simulink model "main_controller_sim"  (R2015a)
settings: Solver=ode45  StartTime=0.0  StopTime=10  FixedStep=1e-4  MaxStep=1e-3  RelTol=1e-3
values from neighbouring files (symbols this model uses):
  A = [-1.27797343778 0.333872204357 1.75620734089 -1.56224484389 -1.03731554325 1.61047691587 -0.301778945187 -0.746429865998 -1.0138823557 1.30543582149 -0.0889326780489 0.0332636291631 ... (36 elements, 6x6)]    [A.mat]    (also in main_Observer.m = sys_rand.A)
  B = [-0.333073072673  -0.110223384653; -0.886176721199  0.948351131026; -0.150737126395  1.10111498524; 0  0.325274480302; 1.26534516191  1.00523432387; 0  0]    [B.mat]    (also in main_Observer.m = B(:,1:end-1))
  C = [0.8954663563 -0.344571536199 -1.3867839766 0 0 -1.25274492024 0.0740580691775 -0.828704014931 -0.552438671582 0 -0.23750602142 -0.378709097599 ... (18 elements, 3x6)]    [C.mat]    (also in main_Observer.m = sys_rand.C)
  Delta = (eye(n,n)+(-H*CHp+Y*(eye(p,p)-(C*H)*CHp))*C)*B    [main_Observer.m]    (also in observer.mat = [1.06190567075  -3.812249351; 850.258941028  448.332221539; )
  Gama = eta*A-X*C    [main_Observer.m]    (also in observer.mat = [22.8246151403 -1331.98593789 -219.710031357 145.030296815 2)
  H = [0.574066719729 0.519875550069 -0.636819062075 -0.770886938571 0.309777205751 -0.804844094201]    [H.mat]    (also in main_Observer.m = B(:,end))
  Phi = inv(delta1)*Phi_hat    [main_Observer.m]    (also in observer.mat = [35.9769844985 416.30041215 22.0641801854 39.341911218 -79.7)
  theta = theta1+Y*theta2    [main_Observer.m]    (also in observer.mat = [0.23961688316 -297.740368665 3.95476908974 -0.24732331029 -)
undefined symbols (not defined in the file or in its folder): beta, Tw, Tx
settings Model: Creator=p4wp4w  LastModifiedBy=p4wp4w

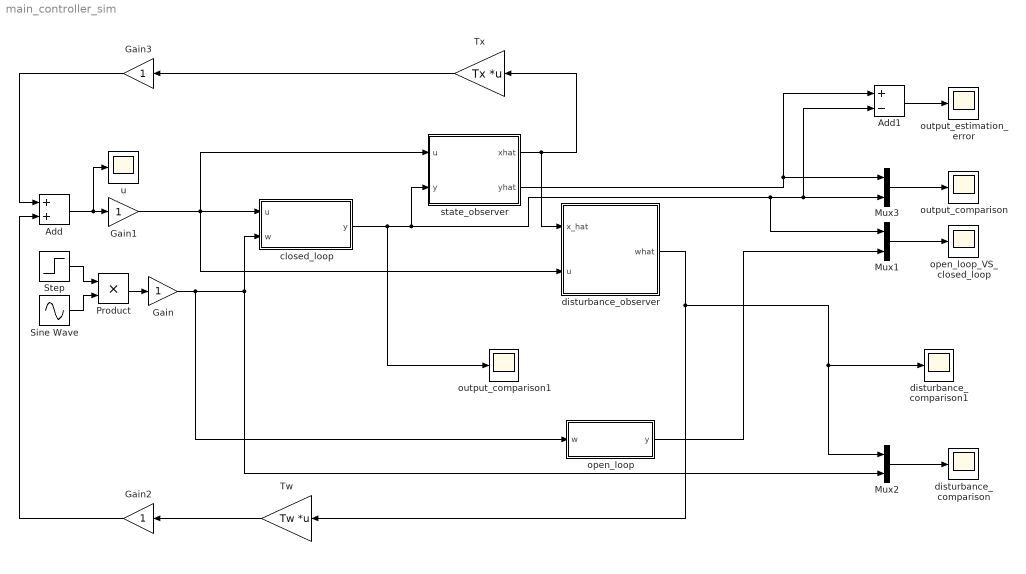
== system main_controller_sim ==
  Add : Sum
  Add1 : Sum  Inputs=+-
  Gain{,1..3} (4 alike) : Gain
  Mux1 : Mux  Inputs=2
  Mux2 : Mux  Inputs=2
  Mux3 : Mux  Inputs=2
  Product : Product
  Sine Wave : Sin  Frequency=10  SampleTime=0
  Step : Step  Before=8  After=0  SampleTime=0
  Tw : Gain  Gain=Tw  Multiplication=Matrix(K*u)
  Tx : Gain  Gain=Tx  Multiplication=Matrix(K*u)
  closed_loop : Subsystem
  disturbance_comparison : Scope
      settings: YMin=-15  YMax=15
  disturbance_comparison1 : Scope
      settings: YMin=-15  YMax=15  SaveName=ScopeData6
  disturbance_observer : Subsystem
  open_loop : Subsystem
  open_loop_VS_closed_loop : Scope
      settings: ShowLegends=on  YMin=-5e+22  YMax=3.5e+23  SaveName=ScopeData4
  output_comparison : Scope
      settings: YMin=-0.0024  YMax=-2.1684e-19
  output_comparison1 : Scope
      settings: YMin=-0.0024  YMax=-2.1684e-19  SaveName=ScopeData5
  output_estimation_error : Scope
      settings: YMin=-0.0024  YMax=-2.1684e-19  SaveName=ScopeData3
  state_observer : Subsystem
  u : Scope
      settings: SaveName=ScopeData2
  wires:
  Gain1/1 -> disturbance_observer/2(u), state_observer/1(u), closed_loop/1(u)
  closed_loop/1(y) -> output_comparison1/1, Mux1/1, Add1/2, Mux3/2, state_observer/2(y)
  Mux2/1 -> disturbance_comparison/1
  Mux3/1 -> output_comparison/1
  state_observer/2(yhat) -> Add1/1, Mux3/1
  disturbance_observer/1(what) -> Tw/1, disturbance_comparison1/1, Mux2/1
  Gain/1 -> open_loop/1(w), Mux2/2, closed_loop/2(w)
  state_observer/1(xhat) -> disturbance_observer/1(x_hat), Tx/1
  Add/1 -> u/1, Gain1/1
  Tx/1 -> Gain3/1
  Tw/1 -> Gain2/1
  Gain2/1 -> Add/2
  Gain3/1 -> Add/1
  Add1/1 -> output_estimation_error/1
  open_loop/1(y) -> Mux1/2
  Mux1/1 -> open_loop_VS_closed_loop/1
  Product/1 -> Gain/1
  Step/1 -> Product/1
  Sine Wave/1 -> Product/2

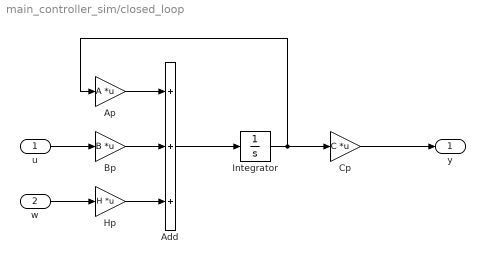
== system main_controller_sim/closed_loop ==
  u : Inport
  w : Inport  Port=2
  Add : Sum  Inputs=+++
  Ap : Gain  Gain=A  Multiplication=Matrix(K*u)
  Bp : Gain  Gain=B  Multiplication=Matrix(K*u)
  Cp : Gain  Gain=C  Multiplication=Matrix(K*u)
  Hp : Gain  Gain=H  Multiplication=Matrix(K*u)
  Integrator : Integrator
  y : Outport
  wires:
  w/1 -> Hp/1
  u/1 -> Bp/1
  Add/1 -> Integrator/1
  Bp/1 -> Add/2
  Integrator/1 -> Cp/1, Ap/1
  Ap/1 -> Add/1
  Hp/1 -> Add/3
  Cp/1 -> y/1

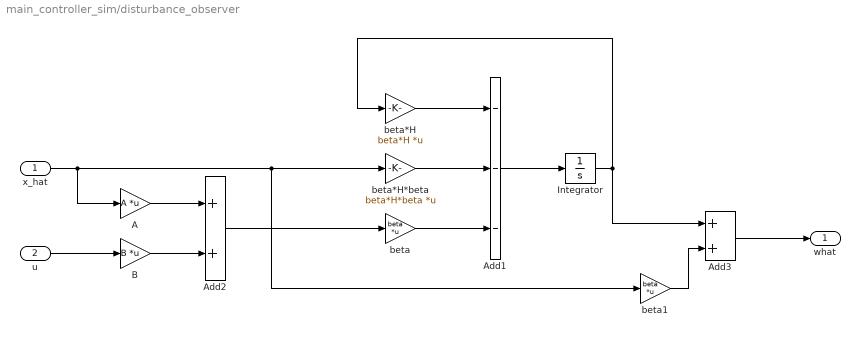
== system main_controller_sim/disturbance_observer ==
  x_hat : Inport
  u : Inport  Port=2
  A : Gain  Gain=A  Multiplication=Matrix(K*u)
  Add1 : Sum  Inputs=---
  Add2 : Sum
  Add3 : Sum
  B : Gain  Gain=B  Multiplication=Matrix(K*u)
  Integrator : Integrator
  beta : Gain  Gain=beta  Multiplication=Matrix(K*u)
  beta*H : Gain  Gain=beta*H  Multiplication=Matrix(K*u)
  beta*H*beta : Gain  Gain=beta*H*beta  Multiplication=Matrix(K*u)
  beta1 : Gain  Gain=beta  Multiplication=Matrix(K*u)
  what : Outport
  wires:
  Add1/1 -> Integrator/1
  beta*H/1 -> Add1/1
  Integrator/1 -> Add3/1, beta*H/1
  beta*H*beta/1 -> Add1/2
  x_hat/1 -> A/1, beta1/1, beta*H*beta/1
  beta/1 -> Add1/3
  A/1 -> Add2/1
  B/1 -> Add2/2
  u/1 -> B/1
  Add2/1 -> beta/1
  beta1/1 -> Add3/2
  Add3/1 -> what/1

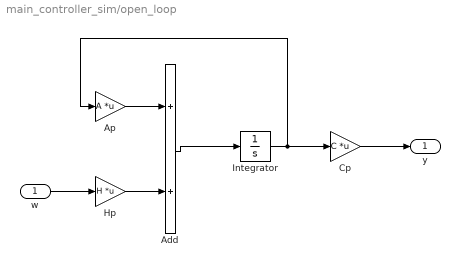
== system main_controller_sim/open_loop ==
  w : Inport
  Add : Sum
  Ap : Gain  Gain=A  Multiplication=Matrix(K*u)
  Cp : Gain  Gain=C  Multiplication=Matrix(K*u)
  Hp : Gain  Gain=H  Multiplication=Matrix(K*u)
  Integrator : Integrator
  y : Outport
  wires:
  Cp/1 -> y/1
  Hp/1 -> Add/2
  Ap/1 -> Add/1
  Integrator/1 -> Ap/1, Cp/1
  Add/1 -> Integrator/1
  w/1 -> Hp/1

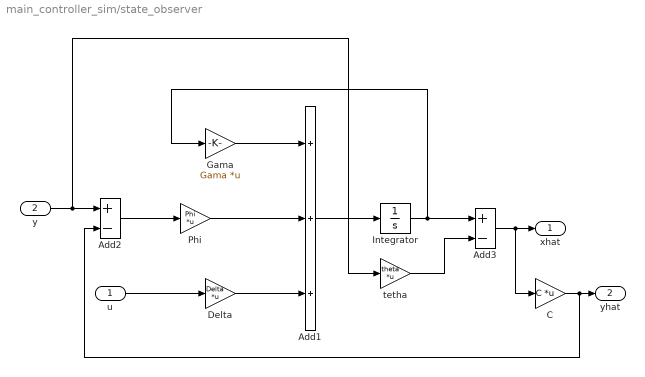
== system main_controller_sim/state_observer ==
  u : Inport
  y : Inport  Port=2
  Add1 : Sum  Inputs=+++
  Add2 : Sum  Inputs=+-
  Add3 : Sum  Inputs=+-
  C : Gain  Gain=C  Multiplication=Matrix(K*u)
  Delta : Gain  Gain=Delta  Multiplication=Matrix(K*u)
  Gama : Gain  Gain=Gama  Multiplication=Matrix(K*u)
  Integrator : Integrator
  Phi : Gain  Gain=Phi  Multiplication=Matrix(K*u)
  tetha : Gain  Gain=theta  Multiplication=Matrix(K*u)
  xhat : Outport
  yhat : Outport  Port=2
  wires:
  y/1 -> tetha/1, Add2/1
  C/1 -> Add2/2, yhat/1
  Add1/1 -> Integrator/1
  Gama/1 -> Add1/1
  Integrator/1 -> Gama/1, Add3/1
  Phi/1 -> Add1/2
  Add2/1 -> Phi/1
  u/1 -> Delta/1
  Delta/1 -> Add1/3
  tetha/1 -> Add3/2
  Add3/1 -> C/1, xhat/1
